simulink model "B2B_HVDC_MMC"  (R2023b)
settings: Solver=ode23t  StartTime=0.0  StopTime=3  FixedStep=Ts_Power  MaxStep=1e-3  MinStep=Ts_Power  RelTol=1e-3
values from neighbouring files (symbols this model uses):
  AC_lim = 1*[1.5 -1.5]    [B2B_HVDC_MMC_Calc.m]
  C_pm = 10.48e-3    (= 0.01048)    [B2B_HVDC_MMC_Calc.m]
  Carm = 1.0*C_pm/n    (= 0.0002096)    [B2B_HVDC_MMC_Calc.m]    (also in HVDC_MMC_param.m = 4.88333333333e-05)
  ccsc_lim = 1*[1.0 -1.0]    [B2B_HVDC_MMC_Calc.m]
  DC_lim = 1*[1.05 -1.05]    [B2B_HVDC_MMC_Calc.m]
  f = 50    [B2B_HVDC_MMC_Calc.m]
  Fn_filter = 1000    [B2B_HVDC_MMC_Calc.m]    (also in HVDC_MMC_param.m)
  Fnom = 50    [HVDC_MMC_param.m]
  HrmOrd = N    (= 2)    [B2B_HVDC_MMC_Calc.m]    (also in HVDC_MMC_param.m)
  I_nom = S_nom/(sqrt(3)*V_grid)    [B2B_HVDC_MMC_Calc.m]
  Ireg_lim_i = 1*[1.5, -1.5]    [B2B_HVDC_MMC_Calc.m]
  Ireg_lim_r = 2*[1.5, -1.5]    [B2B_HVDC_MMC_Calc.m]
  Ki_ACreg_i = 260    [B2B_HVDC_MMC_Calc.m]
  Ki_ccsc = 5    [B2B_HVDC_MMC_Calc.m]
  Ki_DCreg_r = 150    [B2B_HVDC_MMC_Calc.m]
  Ki_Ireg_i = 200    [B2B_HVDC_MMC_Calc.m]
  Ki_Ireg_r = 50    [B2B_HVDC_MMC_Calc.m]
  Kp_ACreg_i = 2    [B2B_HVDC_MMC_Calc.m]
  Kp_ccsc = 1    [B2B_HVDC_MMC_Calc.m]
  Kp_DCreg_r = 8    [B2B_HVDC_MMC_Calc.m]
  Kp_Ireg_i = 2    [B2B_HVDC_MMC_Calc.m]
  Kp_Ireg_r = 0.8    [B2B_HVDC_MMC_Calc.m]
  L1_si = L1_pu*Z_base66/w    [B2B_HVDC_MMC_Calc.m]
  L_arm = L_arm_pu*Z_base66/w    [B2B_HVDC_MMC_Calc.m]
  L_arm_pu = 0.15    [B2B_HVDC_MMC_Calc.m]
  N = 2    [B2B_HVDC_MMC_Calc.m]
  P_nom = 220e6    (= 220000000)    [B2B_HVDC_MMC_Calc.m]
  R1_si = R1_pu*Z_base66    [B2B_HVDC_MMC_Calc.m]
  R_arm = 0.03    [B2B_HVDC_MMC_Calc.m]
  R_arm_pu = R_arm/Z_base66    [B2B_HVDC_MMC_Calc.m]
  R_load = 0.6*40    (= 24)    [B2B_HVDC_MMC_Calc.m]
  R_startup = 17    [B2B_HVDC_MMC_Calc.m]    (also in HVDC_MMC_param.m = 400)
  T_fault = 1.4    [B2B_HVDC_MMC_Calc.m]
  Ts = Ts_Power    (= 5e-05)    [B2B_HVDC_MMC_Calc.m]    (also in HVDC_MMC_param.m)
  Ts_Control = Ts_Power    (= 5e-05)    [B2B_HVDC_MMC_Calc.m]    (also in HVDC_MMC_param.m)
  Ts_DQN = MultTs*Ts_Power    (= 5e-05)    [B2B_HVDC_MMC_Calc.m]    (also in HVDC_MMC_param.m)
  Ts_Power = 1*50e-6    (= 5e-05)    [B2B_HVDC_MMC_Calc.m]    (also in HVDC_MMC_param.m)
  V_ac_ref = 1.035    [B2B_HVDC_MMC_Calc.m]
  V_grid = 66e3    (= 66000)    [B2B_HVDC_MMC_Calc.m]
  Vdc_nom = 135e3    (= 135000)    [B2B_HVDC_MMC_Calc.m]
  Vnom_prim = 333e3    (= 333000)    [HVDC_MMC_param.m]
  Xdcpnz = [zeros(6,1), Xpnz]    [B2B_HVDC_MMC_Calc.m]
  Zeta_filter = 1    [B2B_HVDC_MMC_Calc.m]    (also in HVDC_MMC_param.m)
undefined symbols (not defined in the file or in its folder): DiscIntNeverNeededParam, Pcc, Xdcpnz_c
libraries: DQN_Lib x39, simulink x26, eeTransforms x21, spsCurrentMeasurementLib x16, spsHalfBridgeMMCLib x12, spsSeriesRLCBranchLib x12, B2B_HVDC_MMC_Lib x8, spsSecondOrderFilterLib x8, spsAlphaBetaZerotodq0Lib x6, spsabctoAlphaBetaZeroLib x6, spsThreePhaseVIMeasurementLib x4, spsabctodq0Lib x3
(part 5 of 5)

== matlab function B2B_HVDC_MMC/MMC Converter4/MATLAB Function ==
  data: Ydcpnz_c output; X_DQN input
function Ydcpnz_c  = fDQN012C(X_DQN)
        
            if(size(X_DQN,2) < 1)
                error('Wrong size!');
            end
            
            N = size(X_DQN,1);
        
            if(size(X_DQN,1) == 6 && size(X_DQN,2) == 1)
                N = 1;
                X_DQN = X_DQN';
            end
        
            Ydcpnz_c = complex(zeros(3,N));
        
            for i = 1 : N
             
                if(i>1)
                    Ydcpnz_c(1,i) = (X_DQN(i,1)) + 1i*X_DQN(i,4);
                    Ydcpnz_c(2,i) = (-X_DQN(i,2)) + 1i*X_DQN(i,5);
                    Ydcpnz_c(3,i) = (X_DQN(i,3)) + 1i*X_DQN(i,6);
                else
        
                    Ydcpnz_c(1,i) = 0.5*(X_DQN(i,4) - 1i*X_DQN(i,1));
                    Ydcpnz_c(2,i) = 0.5*(X_DQN(i,5) + 1i*X_DQN(i,2));
                    Ydcpnz_c(3,i) =     (X_DQN(i,6) + 1i*X_DQN(i,3));
                end
            
            end
        
        
end

== matlab function B2B_HVDC_MMC/DQn->ABC ==
  settings: updateMethod=DISCRETE
  data: Xdcpnz_c input; tho input; Xabc output; N parameter
%function abc = Mult(Z0,Zdp,Zqp,Zdn,Zqn,Zdz,Zqz,th, N)
function Xabc = dqn2abc(Xdcpnz_c,tho,N)

    persistent Sas;
    persistent Ssa;

    if(isempty(Sas)) 
        a = -0.5+0.866i;
        a2 = -0.5-0.866i;
        Sas = [1,a,a2;1,a2,a;1,1,1]/3;
        Ssa = eye(3)/(Sas);
    end

    Xabc = zeros(3,1);

    for i = 1 : N+1
    
    
        if(i>1)
            h = i-1;
    
            th = h*tho;
        
            mag_p = abs(Xdcpnz_c(1,i));
            ang_p = angle(Xdcpnz_c(1,i));
            mag_n = abs(Xdcpnz_c(2,i));
            ang_n = angle(Xdcpnz_c(2,i));
            mag_z = abs(Xdcpnz_c(3,i));
            ang_z = angle(Xdcpnz_c(3,i));
            
            abc3p = mag_p*[sin(th+ang_p) ; sin(th+ang_p-2*pi/3) ; sin(th+ang_p+2*pi/3) ];
            abc3n = mag_n*[sin(th+ang_n) ; sin(th+ang_n+2*pi/3) ; sin(th+ang_n-2*pi/3) ];
            abc3z = mag_z*[sin(th+ang_z) ; sin(th+ang_z)        ; sin(th+ang_z)  ];
        
            Xabc = Xabc + abc3p+abc3n+abc3z;
        else
            Xabc = Xabc + real(Ssa*(Xdcpnz_c(:,1)));
        
        end
    
        
    end

end

== matlab function B2B_HVDC_MMC/MATLAB Function8 ==
  data: Xpnz_ci input; Xabc output; tho input; HRM parameter; Xpnz_c output
function [Xabc,Xpnz_c] = fcn(Xpnz_ci, tho, HRM)

Xabc = zeros(3,1);


a = -0.5+0.866i;
a2 = -0.5-0.866i;
Sas = [1,a,a2;1,a2,a;1,1,1]/3;
Ssa = inv(Sas);

for i = 1 : HRM+1


    if(i>1)
        h = i-1;

        th = h*tho;
    
        mag_p = abs(Xpnz_ci(1,i));
        ang_p = angle(Xpnz_ci(1,i));
        mag_n = abs(Xpnz_ci(2,i));
        ang_n = angle(Xpnz_ci(2,i));
        mag_z = abs(Xpnz_ci(3,i));
        ang_z = angle(Xpnz_ci(3,i));
        
        abc3p = mag_p*[sin(th+ang_p) ; sin(th+ang_p-2*pi/3) ; sin(th+ang_p+2*pi/3) ];
        abc3n = mag_n*[sin(th+ang_n) ; sin(th+ang_n+2*pi/3) ; sin(th+ang_n-2*pi/3) ];
        abc3z = mag_z*[sin(th+ang_z) ; sin(th+ang_z)        ; sin(th+ang_z)  ];
    
        Xabc = Xabc + abc3p+abc3n+abc3z;
    else
        Xabc = Xabc + real(Ssa*(Xpnz_ci(:,1)));
    
    end

Xpnz_c = Xpnz_ci;
    
end

== matlab function B2B_HVDC_MMC/MMC Converter2/Int ==
  data: x input; z output; dt parameter
function z  = fcn(x, dt)

    persistent z_old;    
    persistent x_old;   
    persistent dt2;
    
    if(isempty(dt2))
        dt2 = dt/2; 
        z_old  = zeros(3,1);
        x_old  = zeros(3,1);
    end
    
    R = 0.0300;
    iL = 61.0707;
    Krl1 = (dt2*iL/(1+dt2*R*iL));
    Krl2 = (1-dt2*R*iL)/(1+dt2*R*iL);
    
    z = zeros(3,1);

    %z = (dt2)*(x+x_old)+z_old;
    z = Krl1*(x+x_old)+Krl2*z_old;
    z_old = z;
    x_old = x;
    
end

== matlab function B2B_HVDC_MMC/MATLAB Function3 ==
  data: Xpnz input; Xabc output; th input; HRM parameter; X_DQN output; chkHrmLst parameter; HrmLst parameter
function [Xabc, X_DQN] = fcn(Xpnz, th, HRM, chkHrmLst, HrmLst)
abc3p = zeros(3,1);

    X_DQN = zeros((HRM+1)*6,1);
    
    if(chkHrmLst)
        range = numel(HrmLst);
    else
       range = HRM+1; 
       
    end
    
    h = 0;
    for i = 1:range
        
        if(chkHrmLst)
            h = HrmLst(i)+1;
        else
            h = i; 
        end
        
        Magp = Xpnz(1,h);
        Angp = Xpnz(2,h);
        Magn = Xpnz(3,h);
        Angn = Xpnz(4,h);
        Magz = Xpnz(5,h);
        Angz = Xpnz(6,h);

        Xdp = Magp*cos(Angp);
        Xqp = Magp*sin(Angp);
        Xdn =-Magn*cos(Angn);
        Xqn = Magn*sin(Angn);
        Xdz = Magz*cos(Angz);
        Xqz = Magz*sin(Angz);

        Tda_p = [sin((h-1)*th)            cos((h-1)*th);
                 sin((h-1)*th-2*pi/3)     cos((h-1)*th-2*pi/3);
                 sin((h-1)*th+2*pi/3)     cos((h-1)*th+2*pi/3)];

        Tda_n = [sin(-(h-1)*th)           cos(-(h-1)*th);
                 sin(-(h-1)*th-2*pi/3)    cos(-(h-1)*th-2*pi/3);
                 sin(-(h-1)*th+2*pi/3)    cos(-(h-1)*th+2*pi/3)];

        Tda_z = [sin((h-1)*th)            cos((h-1)*th);
                 sin((h-1)*th)            cos((h-1)*th);
                 sin((h-1)*th)            cos((h-1)*th)];


        Tdqn_a = [Tda_p(:,1)  Tda_n(:,1)  Tda_z(:,1)  Tda_p(:,2)  Tda_n(:,2)  Tda_z(:,2)];

        if(h==1)
            abc3p = abc3p + Tdqn_a*[Xdp;-Xdn;Xdz;Xqp;Xqn;Xqz];
            
            X_DQN(h+0*(HRM+1)) = 2*Xdp;
            X_DQN(h+1*(HRM+1)) = -2*Xdn;
            X_DQN(h+2*(HRM+1)) = 0;
            X_DQN(h+3*(HRM+1)) = 2*Xqp;
            X_DQN(h+4*(HRM+1)) = 2*Xqn;
            X_DQN(h+5*(HRM+1)) = Xqz;
            
        else
            abc3p = abc3p + Tdqn_a*[Xdp;Xdn;Xdz;Xqp;Xqn;Xqz];
            
            X_DQN(h+0*(HRM+1)) = Xdp;
            X_DQN(h+1*(HRM+1)) = Xdn;
            X_DQN(h+2*(HRM+1)) = Xdz;
            X_DQN(h+3*(HRM+1)) = Xqp;
            X_DQN(h+4*(HRM+1)) = Xqn;
            X_DQN(h+5*(HRM+1)) = Xqz;
        end
        


    end


    Xabc = abc3p;
    
end

== matlab function B2B_HVDC_MMC/MMC Converter2/Int2 ==
  data: x input; z output; dt parameter
function z = fcn(x, dt)

    persistent z_old;    
    persistent x_old;   
    persistent dt2;
    
    if(isempty(dt2))
        dt2 = dt/2; 
        z_old  = zeros(3,1);
        x_old  = zeros(3,1);
    end
    
    R = 0.0300;
    iL = 61.0707;
    Krl1 = (dt2*iL/(1+dt2*R*iL));
    Krl2 = (1-dt2*R*iL)/(1+dt2*R*iL);
    
    z = zeros(3,1);

    %z = (dt2)*(x+x_old)+z_old;
    z = Krl1*(x+x_old)+Krl2*z_old;
    z_old = z;
    x_old = x;
    
end

== matlab function B2B_HVDC_MMC/MMC Converter4/MATLAB Function1 ==
  data: Ydcpnz_c output; X_DQN input
function Ydcpnz_c  = fDQN012C(X_DQN)
        
            if(size(X_DQN,2) < 1)
                error('Wrong size!');
            end
            
            N = size(X_DQN,1);
        
            if(size(X_DQN,1) == 6 && size(X_DQN,2) == 1)
                N = 1;
                X_DQN = X_DQN';
            end
        
            Ydcpnz_c = complex(zeros(3,N));
        
            for i = 1 : N
             
                if(i>1)
                    Ydcpnz_c(1,i) = (X_DQN(i,1)) + 1i*X_DQN(i,4);
                    Ydcpnz_c(2,i) = (-X_DQN(i,2)) + 1i*X_DQN(i,5);
                    Ydcpnz_c(3,i) = (X_DQN(i,3)) + 1i*X_DQN(i,6);
                else
        
                    Ydcpnz_c(1,i) = 0.5*(X_DQN(i,4) - 1i*X_DQN(i,1));
                    Ydcpnz_c(2,i) = 0.5*(X_DQN(i,5) + 1i*X_DQN(i,2));
                    Ydcpnz_c(3,i) =     (X_DQN(i,6) + 1i*X_DQN(i,3));
                end
            
            end
        
        
end

== matlab function B2B_HVDC_MMC/MMC Converter8/Int ==
  data: x input; z output; dt parameter
function z  = fcn(x, dt)

    persistent z_old;    
    persistent x_old;   
    persistent dt2;
    
    if(isempty(dt2))
        dt2 = dt/2; 
        z_old  = zeros(3,1);
        x_old  = zeros(3,1);
    end
    
    R = 0.0300;
    iL = 61.0707;
    Krl1 = (dt2*iL/(1+dt2*R*iL));
    Krl2 = (1-dt2*R*iL)/(1+dt2*R*iL);
    
    z = zeros(3,1);

    %z = (dt2)*(x+x_old)+z_old;
    z = Krl1*(x+x_old)+Krl2*z_old;
    z_old = z;
    x_old = x;
    
end

== matlab function B2B_HVDC_MMC/MMC Converter8/Int2 ==
  data: x input; z output; dt parameter
function z = fcn(x, dt)

    persistent z_old;    
    persistent x_old;   
    persistent dt2;
    
    if(isempty(dt2))
        dt2 = dt/2; 
        z_old  = zeros(3,1);
        x_old  = zeros(3,1);
    end
    
    R = 0.0300;
    iL = 61.0707;
    Krl1 = (dt2*iL/(1+dt2*R*iL));
    Krl2 = (1-dt2*R*iL)/(1+dt2*R*iL);
    
    z = zeros(3,1);

    %z = (dt2)*(x+x_old)+z_old;
    z = Krl1*(x+x_old)+Krl2*z_old;
    z_old = z;
    x_old = x;
    
end
